simulink model "trabajo_version_antigua"  (R2021a)
settings: Solver=VariableStepAuto  StartTime=0.0  StopTime=1000  RelTol=1e-3
libraries: simulink x2
settings Model: Creator=david  LastModifiedBy=david

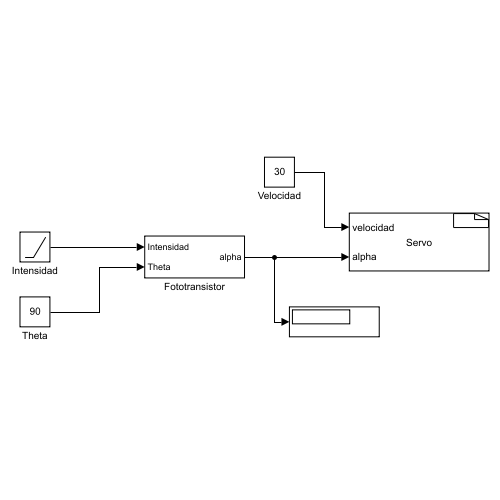
[thumbnail: Simulink's stored preview of the top-level diagram]
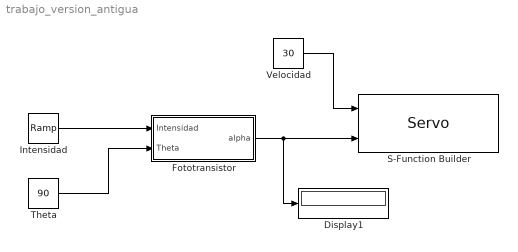
== system trabajo_version_antigua ==
  Display1 : Display
  Fototransistor : Subsystem
  Intensidad : simulink/Sources/Ramp  slope=-0.001  start=0  InitialOutput=1
  S-Function Builder : S-Function  FunctionName=Servo  SFunctionDeploymentMode=off  EnableBusSupport=off  mask(S-Function Builder){}
      mask help: Simulink:masks:SFunctionBuilder_MD
      mask init:
      | val = [[.9  0.75 0.75 1 1 .9 .9 1]',[1 1 0.75 0.75 .9 .9 1 .9]'];try , sys = get_param(gcb,'SfunBuilderFcnName');if isempty(sys), sys = get_param(gcb,'FunctionName'); end,catch, sys = get_param(gcb,'FunctionName'); end
      settings: CopyFcn=set_param(gcbh,'LinkStatus','none')  OpenFcn=sfunctionwizard(gcbh)
      mask Display: plot(val(:,1),val(:,2)),disp(sys),port_label('input',1,'velocidad'),port_label('input',2,'alpha')
  Theta : Constant  Value=90
  Velocidad : Constant  Value=30
  wires:
  Intensidad/1 -> Fototransistor/1(Intensidad)
  Theta/1 -> Fototransistor/2(Theta)
  Fototransistor/1(alpha) -> S-Function Builder/2, Display1/1
  Velocidad/1 -> S-Function Builder/1

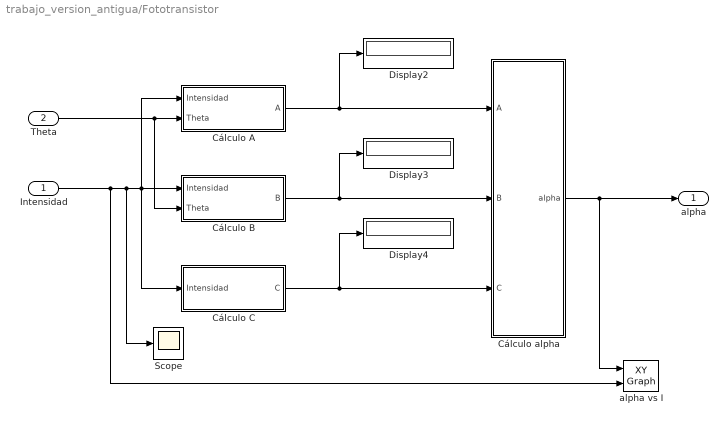
== system trabajo_version_antigua/Fototransistor ==
  Intensidad : Inport
  Theta : Inport  Port=2
  Cálculo A : Subsystem
  Cálculo B : Subsystem
  Cálculo C : Subsystem
  Cálculo alpha : MATLAB Function  TreatAsAtomicUnit=on
  Display2 : Display
  Display3 : Display
  Display4 : Display
  Scope : Scope
  alpha vs I : simulink/Sinks/XY Graph  xmin=-1  xmax=1  ymin=-1  ymax=1  st=-1
  alpha : Outport
  wires:
  Cálculo C/1(C) -> Cálculo alpha/3(C), Display4/1
  Cálculo alpha/1(alpha) -> alpha vs I/1, alpha/1
  Intensidad/1 -> alpha vs I/2, Cálculo C/1(Intensidad), Cálculo B/1(Intensidad), Cálculo A/1(Intensidad), Scope/1
  Theta/1 -> Cálculo B/2(Theta), Cálculo A/2(Theta)
  Cálculo B/1(B) -> Cálculo alpha/2(B), Display3/1
  Cálculo A/1(A) -> Cálculo alpha/1(A), Display2/1

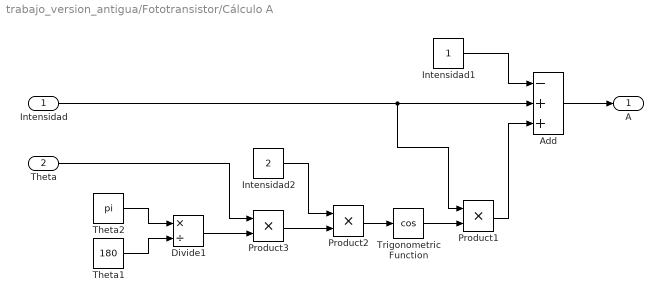
== system trabajo_version_antigua/Fototransistor/Cálculo A ==
  Intensidad : Inport
  Theta : Inport  Port=2
  Add : Sum  Inputs=-++
  Divide1 : Product  Inputs=*/
  Intensidad1 : Constant
  Intensidad2 : Constant  Value=2
  Product1 : Product
  Product2 : Product
  Product3 : Product
  Theta1 : Constant  Value=180
  Theta2 : Constant  Value=pi
  Trigonometric Function : Trigonometry  Operator=cos
  A : Outport
  wires:
  Divide1/1 -> Product3/2
  Product3/1 -> Product2/2
  Theta2/1 -> Divide1/1
  Intensidad1/1 -> Add/1
  Product1/1 -> Add/3
  Theta1/1 -> Divide1/2
  Trigonometric Function/1 -> Product1/2
  Product2/1 -> Trigonometric Function/1
  Intensidad/1 -> Product1/1, Add/2
  Intensidad2/1 -> Product2/1
  Theta/1 -> Product3/1
  Add/1 -> A/1

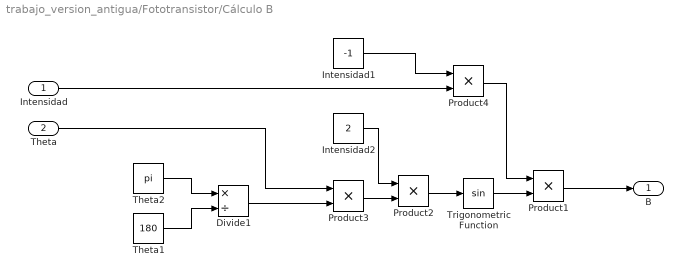
== system trabajo_version_antigua/Fototransistor/Cálculo B ==
  Intensidad : Inport
  Theta : Inport  Port=2
  Divide1 : Product  Inputs=*/
  Intensidad1 : Constant  Value=-1
  Intensidad2 : Constant  Value=2
  Product{1..4} (4 alike) : Product
  Theta1 : Constant  Value=180
  Theta2 : Constant  Value=pi
  Trigonometric Function : Trigonometry
  B : Outport
  wires:
  Divide1/1 -> Product3/2
  Product3/1 -> Product2/2
  Theta2/1 -> Divide1/1
  Product1/1 -> B/1
  Theta1/1 -> Divide1/2
  Trigonometric Function/1 -> Product1/2
  Product2/1 -> Trigonometric Function/1
  Intensidad/1 -> Product4/2
  Intensidad2/1 -> Product2/1
  Theta/1 -> Product3/1
  Intensidad1/1 -> Product4/1
  Product4/1 -> Product1/1

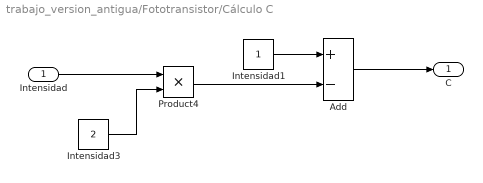
== system trabajo_version_antigua/Fototransistor/Cálculo C ==
  Intensidad : Inport
  Add : Sum  Inputs=+-
  Intensidad1 : Constant
  Intensidad3 : Constant  Value=2
  Product4 : Product
  C : Outport
  wires:
  Intensidad1/1 -> Add/1
  Add/1 -> C/1
  Intensidad/1 -> Product4/1
  Intensidad3/1 -> Product4/2
  Product4/1 -> Add/2

== matlab function trabajo_version_antigua/Fototransistor/Cálculo alpha ==
  data: A input; alpha output; B input; C input
function alpha = fcn(A, B, C)

    if ((A+C ~= 0) && (-B*sqrt(A^2+B^2-C^2)+A^2+A*C+B^2 ~= 0))
        
        alpha = atan((B-sqrt(A^2+B^2-C^2))/(A+C));

    elseif ((A+C ~= 0) && (B*sqrt(A^2+B^2-C^2)+A^2+A*C+B^2 ~= 0))

        alpha = atan((B+sqrt(A^2+B^2-C^2))/(A+C));

    elseif ((B ~= 0) && (A^2+B^2~=0) && (C == -A))

        alpha = -atan(A/B);

    elseif (A == -C)

        alpha = pi/2;

    else

        alpha = 1000;

    end

    alpha = alpha*180/pi;

end
